simulink model "W03_TrafficLight"  (R2020a)
settings: Solver=VariableStepAuto  StartTime=0.0  StopTime=150  RelTol=1e-3
undefined symbols (not defined in the file): DiscIntNeverNeededParam
libraries: simulink x1
settings Model: Creator=Shivam  LastModifiedBy=Shivam

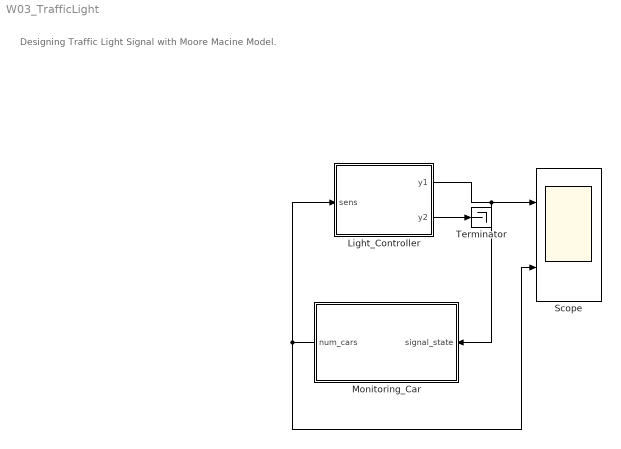
== system W03_TrafficLight ==
  note: Designing Traffic Light Signal
      | with Moore Macine Model.
  Light_Controller : Stateflow chart  TreatAsAtomicUnit=on
  Monitoring_Car : Subsystem
  Scope : Scope  NumInputPorts=2
  Terminator : Terminator
  wires:
  Light_Controller/1(y1) -> Monitoring_Car/1(signal_state), Scope/1
  Monitoring_Car/1(num_cars) -> Light_Controller/1(sens), Scope/2
  Light_Controller/2(y2) -> Terminator/1

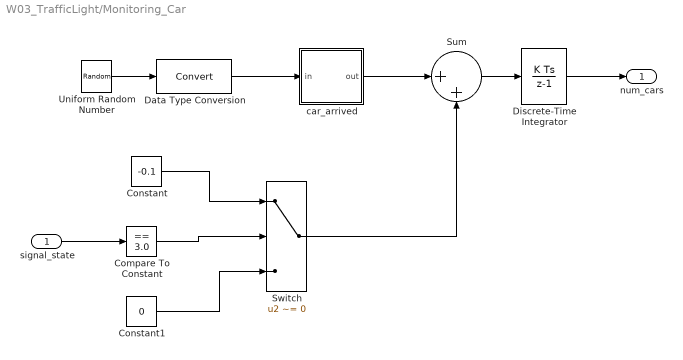
== system W03_TrafficLight/Monitoring_Car ==
  signal_state : Inport
  Compare To Constant : simulink/Logic and Bit Operations/Compare To Constant  relop===  const=3.0  OutDataTypeStr=boolean
  Constant : Constant  Value=-0.1
  Constant1 : Constant  Value=0
  Data Type Conversion : DataTypeConversion
  Discrete-Time Integrator : DiscreteIntegrator  SampleTime=-1  ICPrevOutput=DiscIntNeverNeededParam  ICPrevScaledInput=DiscIntNeverNeededParam
  Sum : Sum  Inputs=|++
  Switch : Switch  Criteria=u2 ~= 0
  Uniform Random Number : UniformRandomNumber  Minimum=0  Maximum=100  Seed=177836  SampleTime=0.1
  car_arrived : Stateflow chart  TreatAsAtomicUnit=on
  num_cars : Outport
  wires:
  Uniform Random Number/1 -> Data Type Conversion/1
  Data Type Conversion/1 -> car_arrived/1(in)
  signal_state/1 -> Compare To Constant/1
  Compare To Constant/1 -> Switch/2
  Constant/1 -> Switch/1
  Constant1/1 -> Switch/3
  car_arrived/1(out) -> Sum/1
  Switch/1 -> Sum/2
  Sum/1 -> Discrete-Time Integrator/1
  Discrete-Time Integrator/1 -> num_cars/1

== stateflow chart W03_TrafficLight/Light_Controller ==
  state Stop
    y1 = RED;
    y2 = GREEN;
  state StopForTraffic
    y1 = RED;
    y2= GREEN;
  state StopToGo
    y1 = RED;
    y2 = YELLOW;
  state GoToStop
    y1 = YELLOW;
    y2 = RED;
  state Go
    y1 = GREEN;
    y2 = RED;
  (default) -> Stop
  Stop -> StopForTraffic : after(20,tick)
  StopForTraffic -> StopToGo : [sens]
  GoToStop -> Stop : after(3,tick)
  StopToGo -> Go : after(3,tick)
  Go -> GoToStop : after(10,tick)
  data: y1 output double; y2 output double; sens input double; RED constant uint8 =1; YELLOW constant double =2; GREEN constant double =3

== stateflow chart W03_TrafficLight/Monitoring_Car/car_arrived ==
  (default) -> (junction 3) : {out = in>98;}
  data: in input; out output
